simulink model "untitled2"  (R2024b)
settings: Solver=VariableStepAuto  StartTime=0.0  StopTime=30  RelTol=1e-3
settings Model: Creator=Corné  LastModifiedBy=Corné

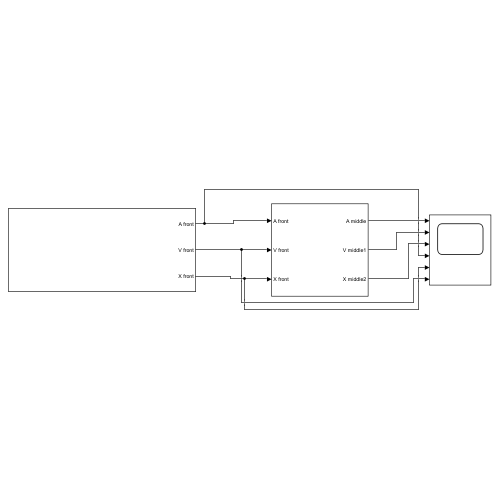
[thumbnail: Simulink's stored preview of the top-level diagram]
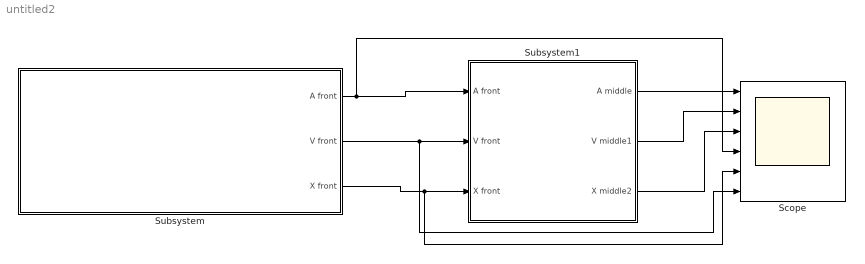
== system untitled2 ==
  Scope : Scope  NumInputPorts=6
  Subsystem : Subsystem
  Subsystem1 : Subsystem
  wires:
  Subsystem/1(A front) -> Scope/4, Subsystem1/1(A front)
  Subsystem/2(V front) -> Scope/6, Subsystem1/2(V front)
  Subsystem/3(X front) -> Scope/5, Subsystem1/3(X front)
  Subsystem1/1(A middle) -> Scope/1
  Subsystem1/2(V middle1) -> Scope/2
  Subsystem1/3(X middle2) -> Scope/3

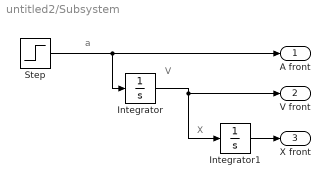
== system untitled2/Subsystem ==
  note: X
  note: V
  note: a
  Integrator : Integrator  InitialCondition=5
  Integrator1 : Integrator
  Step : Step  Time=0  After=0  SampleTime=0
  A front : Outport
  V front : Outport  Port=2
  X front : Outport  Port=3
  wires:
  Integrator/1 -> V front/1, Integrator1/1
  Step/1 -> A front/1, Integrator/1
  Integrator1/1 -> X front/1

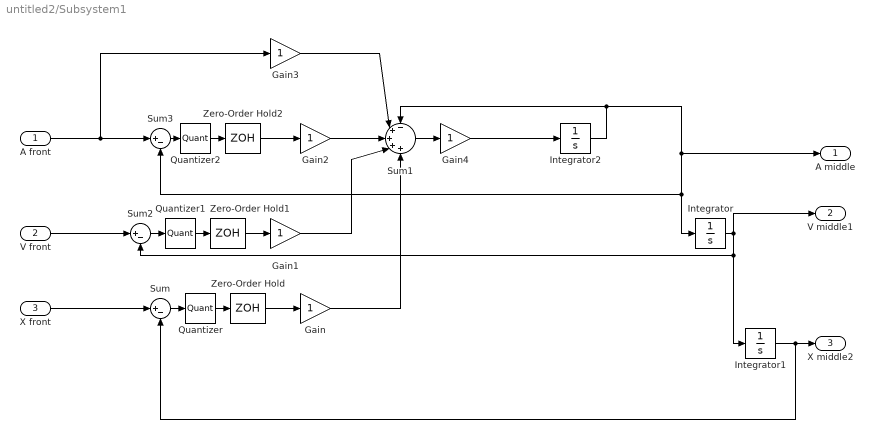
== system untitled2/Subsystem1 ==
  A front : Inport
  V front : Inport  Port=2
  X front : Inport  Port=3
  Gain{,1..4} (5 alike) : Gain
  Integrator : Integrator
  Integrator1 : Integrator
  Integrator2 : Integrator
  Quantizer : Quantizer
  Quantizer1 : Quantizer
  Quantizer2 : Quantizer
  Sum : Sum  Inputs=|+-
  Sum1 : Sum  Inputs=-++++
  Sum2 : Sum  Inputs=|+-
  Sum3 : Sum  Inputs=|+-
  Zero-Order Hold : ZeroOrderHold  SampleTime=-1
  Zero-Order Hold1 : ZeroOrderHold  SampleTime=-1
  Zero-Order Hold2 : ZeroOrderHold  SampleTime=-1
  A middle : Outport
  V middle1 : Outport  Port=2
  X middle2 : Outport  Port=3
  wires:
  Integrator2/1 -> Integrator/1, Sum3/2, A middle/1, Sum1/1
  Integrator/1 -> V middle1/1, Integrator1/1, Sum2/2
  Integrator1/1 -> X middle2/1, Sum/2
  X front/1 -> Sum/1
  Sum/1 -> Quantizer/1
  Quantizer/1 -> Zero-Order Hold/1
  Zero-Order Hold/1 -> Gain/1
  V front/1 -> Sum2/1
  Sum2/1 -> Quantizer1/1
  Quantizer1/1 -> Zero-Order Hold1/1
  Zero-Order Hold1/1 -> Gain1/1
  A front/1 -> Gain3/1, Sum3/1
  Sum3/1 -> Quantizer2/1
  Quantizer2/1 -> Zero-Order Hold2/1
  Zero-Order Hold2/1 -> Gain2/1
  Gain3/1 -> Sum1/2
  Gain2/1 -> Sum1/3
  Gain/1 -> Sum1/5
  Gain1/1 -> Sum1/4
  Gain4/1 -> Integrator2/1
  Sum1/1 -> Gain4/1
